simulink model "debug_seesawIMU_legacy"  (Simulink 8.3)
settings: Solver=FixedStepDiscrete  StartTime=0.0  StopTime=inf  FixedStep=0.01  RelTol=1e-3
libraries: WBToolboxLibrary x2
settings Model: Creator=The MathWorks, Inc.  LastModifiedBy=gnava
settings DataIOCC: SaveFormat=StructureWithTime  SignalLoggingSaveFormat=Dataset
settings DebuggingCC: UnderspecifiedInitializationDetection=Simplified  MergeDetectMultiDrivingBlocksExec=error  SolverPrmCheckMsg=none  FrameProcessingCompatibilityMsg=error  StateNameClashWarn=none
settings HardwareCC: ProdBitPerPointer=64  ProdLargestAtomicFloat=Float  ProdIntDivRoundTo=Zero  ProdEndianess=LittleEndian  ProdHWDeviceType=Specified
settings GRTTargetCC: GeneratePreprocessorConditionals=Use local settings  CombineOutputUpdateFcns=on  GRTInterface=off

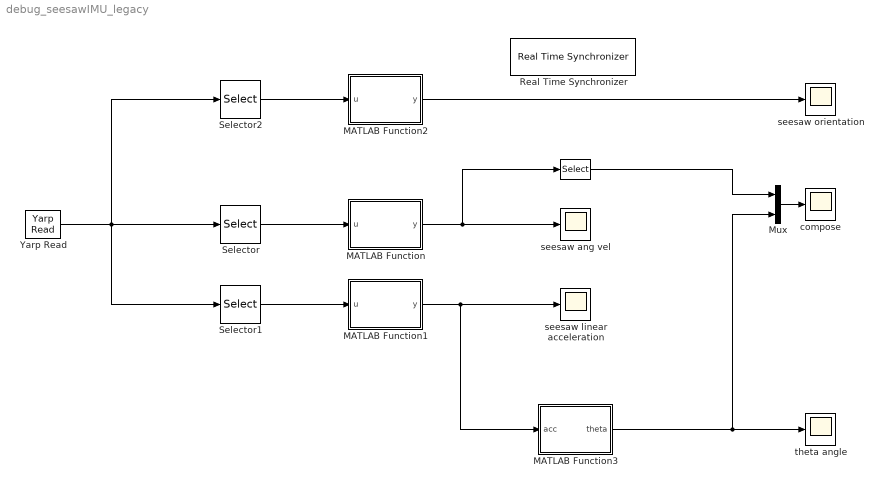
== system debug_seesawIMU_legacy ==
  " " : Selector  InputPortWidth=3  IndexOptions=Index vector (dialog)  Indices=[1]  OutputSizes=1
  MATLAB Function : MATLAB Function  TreatAsAtomicUnit=on
      settings: PermitHierarchicalResolution=ParametersOnly
  MATLAB Function1 : MATLAB Function  TreatAsAtomicUnit=on
      settings: PermitHierarchicalResolution=ParametersOnly
  MATLAB Function2 : MATLAB Function  TreatAsAtomicUnit=on
      settings: PermitHierarchicalResolution=ParametersOnly
  MATLAB Function3 : MATLAB Function  TreatAsAtomicUnit=on
      settings: PermitHierarchicalResolution=ParametersOnly
  Mux : Mux  Inputs=2
  Real Time Synchronizer : WBToolboxLibrary/Utilities/Real Time Synchronizer  period=0.01
  Selector : Selector  InputPortWidth=9  IndexOptions=Index vector (dialog)  Indices=[7 8 9]  OutputSizes=1
  Selector1 : Selector  InputPortWidth=9  IndexOptions=Index vector (dialog)  Indices=[4 5 6]  OutputSizes=1
  Selector2 : Selector  InputPortWidth=9  IndexOptions=Index vector (dialog)  Indices=[1 2 3]  OutputSizes=1
  Yarp Read : WBToolboxLibrary/Utilities/Yarp Read  portName='/seesaw'  signalSize=9  timeout=0.5  blocking=off  timestamp=off  autoconnect=on  errorOnConnection=on
  compose : Scope
      settings: TimeRange=auto  LimitDataPoints=on  MaxDataPoints=5000  SaveToWorkspace=off  SaveName=ScopeData  YMin=-10  YMax=10  SampleTime=-1  DataFormat=Array
  seesaw ang vel : Scope
      settings: TimeRange=auto  LimitDataPoints=on  MaxDataPoints=5000  SaveToWorkspace=off  SaveName=ScopeData  YMin=-10  YMax=10  SampleTime=-1  DataFormat=Array
  seesaw linear acceleration : Scope
      settings: TimeRange=auto  LimitDataPoints=on  MaxDataPoints=5000  SaveToWorkspace=off  SaveName=ScopeData  YMin=-10  YMax=10  SampleTime=-1  DataFormat=Array
  seesaw orientation : Scope
      settings: TimeRange=auto  LimitDataPoints=on  MaxDataPoints=5000  SaveToWorkspace=off  SaveName=ScopeData  YMin=-10  YMax=10  SampleTime=-1  DataFormat=Array
  theta angle : Scope
      settings: TimeRange=auto  LimitDataPoints=on  MaxDataPoints=5000  SaveToWorkspace=off  SaveName=ScopeData  YMin=-10  YMax=10  SampleTime=-1  DataFormat=Array
  wires:
  Yarp Read/1 -> Selector1/1, Selector2/1, Selector/1
  Selector/1 -> MATLAB Function/1(u)
  MATLAB Function/1(y) -> " "/1, seesaw ang vel/1
  Selector1/1 -> MATLAB Function1/1(u)
  MATLAB Function1/1(y) -> seesaw linear acceleration/1, MATLAB Function3/1(acc)
  Selector2/1 -> MATLAB Function2/1(u)
  MATLAB Function2/1(y) -> seesaw orientation/1
  Mux/1 -> compose/1
  MATLAB Function3/1(theta) -> theta angle/1, Mux/2
  " "/1 -> Mux/1

== matlab function MATLAB Function1 ==
  data: u input double; y output double
function y = rotate(u)

y = rotx(pi)*rotz(-44/180*pi)*u;

end

== matlab function MATLAB Function ==
  data: u input double; y output double
function y = rotate(u)

y = rotx(pi)*rotz(-44/180*pi)*u;

end

== matlab function MATLAB Function2 ==
  data: u input double; y output double
function y = rotate(u)

y = rotx(pi)*rotz(-44/180*pi)*u;

end

== matlab function MATLAB Function3 ==
  data: acc input double; theta output double
function theta = arctangent(acc)

theta = atan2(acc(2),acc(3))*180/pi;

end
